simulink model "IOT_Charger"  (R2024b)
settings: Solver=ode23tb  StartTime=0.0  StopTime=1  RelTol=1e-3  EnableMultiTasking=on
PreLoadFcn:
  | % Data of Solar Panel
  | %5000[W]/130[W]
  | % Total power generated by solar panel reaches 5[KW].
  | % each solar panel generates power 130[kW].
  | V = [0    40 80 120 160 180 200 217 240 260 280];
  | I = 5000/130*[0.68 0.675 0.67 0.665 0.660 0.655 0.640 0.6 0.48 0.28 0];
  | 
  | %subplot(211);plot(V,I);xlabel('Voltage[V]');ylabel('Current[a]')
  | %subplot(212);plot(V.*I);title('Power[W]')
  | 
  | % Sample Time[s]
  | Ts =5e-6;
  | 
  | 
  | %MPPT + PV Control
  | % PI control pamameter of Voltage control(Outer loop)
  | Kp_V = 50e-3;
  | Ki_V = 10;
  | 
  | % PI Control pamameter of Current control(Inner loop)
  | Kp_I = 25e-3;
  | Ki_I = 10;
  | 
  | % Utility Interconnection Control
  | % PI Control pamameter of Voltage control(Outer loop)
  | Kp_V2 = 0.01;
  | Ki_V2 = 25;
  | 
  | % PI control pamameter of Current control(Inner loop)
  | Kp_I2 = 0.01;
  | Ki_I2 = 25;
  | 
  | 
  | % Difference of voltege using in MPPT
  | dV = 0.5;
  | 
  | % Battery Control
  | % PI Control pamameter of Voltage control(Outer loop)
  | Kp_VB = 0.4;
  | Ki_VB = 2;
  | 
  | % PI control pamameter of Current control(Inner loop)
  | Kp_IB = 0.1;
  | Ki_IB = 0.5;
undefined symbols (not defined in the file): Ion, Lithium, sigbuilder_block
libraries: spsBreakerLib x120, spsSeriesRLCBranchLib x72, spsBatteryLib x43, spsIdealSwitchLib x29, spsVoltageMeasurementLib x25, spsMosfetLib x19, slpidlib x17, spsSeriesRLCLoadLib x12, spsPWMGeneratorDCDCLib x11, spsCurrentMeasurementLib x10, spsDiodeLib x6, spsPWMGenerator2LevelLib x5
(part 3 of 6)

== system IOT_Charger/Subsystem18/Subsystem20 ==
  Battery : spsBatteryLib/Battery  BatType=Lithium-Ion  NomV=12  NomQ=10  SOC=95  Batt_Tr=30  PresetModel=on  MaxQ=10  MinV=9  FullV=13.9678  Dis_rate=4.3478  R=0.012  Normal_OP=9.0435  expZone="[12.9646     0.491304]"
  Breaker{,1..3} (4 alike) : spsBreakerLib/Breaker  InitialState=0  SwitchingTimes="[1/60  5/60]"  External=on  BreakerResistance=0.01  SnubberResistance=1e6  SnubberCapacitance=inf  Measurements=None  MoreParameters=on  NoBreakLoop=off
  Bus Selector : BusSelector  OutputSignals=SOC (%),Current (A),Voltage (V)
  Scope : Scope  NumInputPorts=3
  Series RLC Branch : spsSeriesRLCBranchLib/Series RLC Branch  LConnTagsString=__new0  RConnTagsString=__new0  BranchType=R  Resistance=1  Inductance=1e-3  SetiL0=off  InitialCurrent=0  Capacitance=1e-6  Setx0=off  InitialVoltage=0  Measurements=None
  + : PMIOPort  Side=Right
  - : PMIOPort  Port=2  Side=Right
  tag scope: s8=global
  wires:
  Battery/1 -> Bus Selector/1
  [c8] -> Breaker3/1, Breaker/1
  Bus Selector/2 -> Scope/2  "<Current (A)>"
  [d8] -> Breaker1/1, Breaker2/1
  Bus Selector/3 -> Scope/3  "<Voltage (V)>"
  Bus Selector/1 -> [s8], Scope/1  "<SOC (%)>"
  connections:
  Breaker2/LConn1 -- Breaker3/RConn1 -- Battery/LConn2
  Breaker1/LConn1 -- Battery/LConn1 -- Breaker/RConn1
  +/RConn1 -- Breaker/LConn1
  Series RLC Branch/LConn1 -- Breaker2/RConn1
  Series RLC Branch/RConn1 -- Breaker1/RConn1
  -/RConn1 -- Breaker3/LConn1

== system IOT_Charger/Subsystem18/Subsystem21 ==
  Battery : spsBatteryLib/Battery  BatType=Lithium-Ion  NomV=12  NomQ=10  SOC=95  Batt_Tr=30  PresetModel=on  MaxQ=10  MinV=9  FullV=13.9678  Dis_rate=4.3478  R=0.012  Normal_OP=9.0435  expZone="[12.9646     0.491304]"
  Breaker{,1..3} (4 alike) : spsBreakerLib/Breaker  InitialState=0  SwitchingTimes="[1/60  5/60]"  External=on  BreakerResistance=0.01  SnubberResistance=1e6  SnubberCapacitance=inf  Measurements=None  MoreParameters=on  NoBreakLoop=off
  Bus Selector : BusSelector  OutputSignals=SOC (%),Current (A),Voltage (V)
  Scope : Scope  NumInputPorts=3
  Series RLC Branch : spsSeriesRLCBranchLib/Series RLC Branch  LConnTagsString=__new0  RConnTagsString=__new0  BranchType=R  Resistance=1  Inductance=1e-3  SetiL0=off  InitialCurrent=0  Capacitance=1e-6  Setx0=off  InitialVoltage=0  Measurements=None
  + : PMIOPort  Side=Right
  - : PMIOPort  Port=2  Side=Right
  tag scope: s7=global
  wires:
  Battery/1 -> Bus Selector/1
  [c7] -> Breaker3/1, Breaker/1
  Bus Selector/2 -> Scope/2  "<Current (A)>"
  [d7] -> Breaker1/1, Breaker2/1
  Bus Selector/3 -> Scope/3  "<Voltage (V)>"
  Bus Selector/1 -> [s7], Scope/1  "<SOC (%)>"
  connections:
  Breaker2/LConn1 -- Breaker3/RConn1 -- Battery/LConn2
  Breaker1/LConn1 -- Battery/LConn1 -- Breaker/RConn1
  +/RConn1 -- Breaker/LConn1
  Series RLC Branch/LConn1 -- Breaker2/RConn1
  Series RLC Branch/RConn1 -- Breaker1/RConn1
  -/RConn1 -- Breaker3/LConn1

== system IOT_Charger/Subsystem18/Subsystem22 ==
  Battery : spsBatteryLib/Battery  BatType=Lithium-Ion  NomV=12  NomQ=10  SOC=95  Batt_Tr=30  PresetModel=on  MaxQ=10  MinV=9  FullV=13.9678  Dis_rate=4.3478  R=0.012  Normal_OP=9.0435  expZone="[12.9646     0.491304]"
  Breaker{,1..3} (4 alike) : spsBreakerLib/Breaker  InitialState=0  SwitchingTimes="[1/60  5/60]"  External=on  BreakerResistance=0.01  SnubberResistance=1e6  SnubberCapacitance=inf  Measurements=None  MoreParameters=on  NoBreakLoop=off
  Bus Selector : BusSelector  OutputSignals=SOC (%),Current (A),Voltage (V)
  Scope : Scope  NumInputPorts=3
  Series RLC Branch : spsSeriesRLCBranchLib/Series RLC Branch  LConnTagsString=__new0  RConnTagsString=__new0  BranchType=R  Resistance=1  Inductance=1e-3  SetiL0=off  InitialCurrent=0  Capacitance=1e-6  Setx0=off  InitialVoltage=0  Measurements=None
  + : PMIOPort  Side=Right
  - : PMIOPort  Port=2  Side=Right
  tag scope: s29=global
  wires:
  Battery/1 -> Bus Selector/1
  [c29] -> Breaker3/1, Breaker/1
  Bus Selector/2 -> Scope/2  "<Current (A)>"
  [d29] -> Breaker1/1, Breaker2/1
  Bus Selector/3 -> Scope/3  "<Voltage (V)>"
  Bus Selector/1 -> [s29], Scope/1  "<SOC (%)>"
  connections:
  Breaker2/LConn1 -- Breaker3/RConn1 -- Battery/LConn2
  Breaker1/LConn1 -- Battery/LConn1 -- Breaker/RConn1
  +/RConn1 -- Breaker/LConn1
  Series RLC Branch/LConn1 -- Breaker2/RConn1
  Series RLC Branch/RConn1 -- Breaker1/RConn1
  -/RConn1 -- Breaker3/LConn1

== system IOT_Charger/Subsystem18/Subsystem23 ==
  Battery : spsBatteryLib/Battery  BatType=Lithium-Ion  NomV=12  NomQ=10  SOC=95  Batt_Tr=30  PresetModel=on  MaxQ=10  MinV=9  FullV=13.9678  Dis_rate=4.3478  R=0.012  Normal_OP=9.0435  expZone="[12.9646     0.491304]"
  Breaker{,1..3} (4 alike) : spsBreakerLib/Breaker  InitialState=0  SwitchingTimes="[1/60  5/60]"  External=on  BreakerResistance=0.01  SnubberResistance=1e6  SnubberCapacitance=inf  Measurements=None  MoreParameters=on  NoBreakLoop=off
  Bus Selector : BusSelector  OutputSignals=SOC (%),Current (A),Voltage (V)
  Scope : Scope  NumInputPorts=3
  Series RLC Branch : spsSeriesRLCBranchLib/Series RLC Branch  LConnTagsString=__new0  RConnTagsString=__new0  BranchType=R  Resistance=1  Inductance=1e-3  SetiL0=off  InitialCurrent=0  Capacitance=1e-6  Setx0=off  InitialVoltage=0  Measurements=None
  + : PMIOPort  Side=Right
  - : PMIOPort  Port=2  Side=Right
  tag scope: s30=global
  wires:
  Battery/1 -> Bus Selector/1
  [c30] -> Breaker3/1, Breaker/1
  Bus Selector/2 -> Scope/2  "<Current (A)>"
  [d30] -> Breaker1/1, Breaker2/1
  Bus Selector/3 -> Scope/3  "<Voltage (V)>"
  Bus Selector/1 -> [s30], Scope/1  "<SOC (%)>"
  connections:
  Breaker2/LConn1 -- Breaker3/RConn1 -- Battery/LConn2
  Breaker1/LConn1 -- Battery/LConn1 -- Breaker/RConn1
  +/RConn1 -- Breaker/LConn1
  Series RLC Branch/LConn1 -- Breaker2/RConn1
  Series RLC Branch/RConn1 -- Breaker1/RConn1
  -/RConn1 -- Breaker3/LConn1

== system IOT_Charger/Subsystem18/Subsystem24 ==
  Battery : spsBatteryLib/Battery  BatType=Lithium-Ion  NomV=12  NomQ=10  SOC=95  Batt_Tr=30  PresetModel=on  MaxQ=10  MinV=9  FullV=13.9678  Dis_rate=4.3478  R=0.012  Normal_OP=9.0435  expZone="[12.9646     0.491304]"
  Breaker{,1..3} (4 alike) : spsBreakerLib/Breaker  InitialState=0  SwitchingTimes="[1/60  5/60]"  External=on  BreakerResistance=0.01  SnubberResistance=1e6  SnubberCapacitance=inf  Measurements=None  MoreParameters=on  NoBreakLoop=off
  Bus Selector : BusSelector  OutputSignals=SOC (%),Current (A),Voltage (V)
  Scope : Scope  NumInputPorts=3
  Series RLC Branch : spsSeriesRLCBranchLib/Series RLC Branch  LConnTagsString=__new0  RConnTagsString=__new0  BranchType=R  Resistance=1  Inductance=1e-3  SetiL0=off  InitialCurrent=0  Capacitance=1e-6  Setx0=off  InitialVoltage=0  Measurements=None
  + : PMIOPort  Side=Right
  - : PMIOPort  Port=2  Side=Right
  tag scope: s26=global
  wires:
  Battery/1 -> Bus Selector/1
  [c26] -> Breaker3/1, Breaker/1
  Bus Selector/2 -> Scope/2  "<Current (A)>"
  [d26] -> Breaker1/1, Breaker2/1
  Bus Selector/3 -> Scope/3  "<Voltage (V)>"
  Bus Selector/1 -> [s26], Scope/1  "<SOC (%)>"
  connections:
  Breaker2/LConn1 -- Breaker3/RConn1 -- Battery/LConn2
  Breaker1/LConn1 -- Battery/LConn1 -- Breaker/RConn1
  +/RConn1 -- Breaker/LConn1
  Series RLC Branch/LConn1 -- Breaker2/RConn1
  Series RLC Branch/RConn1 -- Breaker1/RConn1
  -/RConn1 -- Breaker3/LConn1

== system IOT_Charger/Subsystem18/Subsystem25 ==
  Battery : spsBatteryLib/Battery  BatType=Lithium-Ion  NomV=12  NomQ=10  SOC=95  Batt_Tr=30  PresetModel=on  MaxQ=10  MinV=9  FullV=13.9678  Dis_rate=4.3478  R=0.012  Normal_OP=9.0435  expZone="[12.9646     0.491304]"
  Breaker{,1..3} (4 alike) : spsBreakerLib/Breaker  InitialState=0  SwitchingTimes="[1/60  5/60]"  External=on  BreakerResistance=0.01  SnubberResistance=1e6  SnubberCapacitance=inf  Measurements=None  MoreParameters=on  NoBreakLoop=off
  Bus Selector : BusSelector  OutputSignals=SOC (%),Current (A),Voltage (V)
  Scope : Scope  NumInputPorts=3
  Series RLC Branch : spsSeriesRLCBranchLib/Series RLC Branch  LConnTagsString=__new0  RConnTagsString=__new0  BranchType=R  Resistance=1  Inductance=1e-3  SetiL0=off  InitialCurrent=0  Capacitance=1e-6  Setx0=off  InitialVoltage=0  Measurements=None
  + : PMIOPort  Side=Right
  - : PMIOPort  Port=2  Side=Right
  tag scope: s28=global
  wires:
  Battery/1 -> Bus Selector/1
  [c28] -> Breaker3/1, Breaker/1
  Bus Selector/2 -> Scope/2  "<Current (A)>"
  [d28] -> Breaker1/1, Breaker2/1
  Bus Selector/3 -> Scope/3  "<Voltage (V)>"
  Bus Selector/1 -> [s28], Scope/1  "<SOC (%)>"
  connections:
  Breaker2/LConn1 -- Breaker3/RConn1 -- Battery/LConn2
  Breaker1/LConn1 -- Battery/LConn1 -- Breaker/RConn1
  +/RConn1 -- Breaker/LConn1
  Series RLC Branch/LConn1 -- Breaker2/RConn1
  Series RLC Branch/RConn1 -- Breaker1/RConn1
  -/RConn1 -- Breaker3/LConn1

== system IOT_Charger/Subsystem18/Subsystem26 ==
  Battery : spsBatteryLib/Battery  BatType=Lithium-Ion  NomV=12  NomQ=10  SOC=95  Batt_Tr=30  PresetModel=on  MaxQ=10  MinV=9  FullV=13.9678  Dis_rate=4.3478  R=0.012  Normal_OP=9.0435  expZone="[12.9646     0.491304]"
  Breaker{,1..3} (4 alike) : spsBreakerLib/Breaker  InitialState=0  SwitchingTimes="[1/60  5/60]"  External=on  BreakerResistance=0.01  SnubberResistance=1e6  SnubberCapacitance=inf  Measurements=None  MoreParameters=on  NoBreakLoop=off
  Bus Selector : BusSelector  OutputSignals=SOC (%),Current (A),Voltage (V)
  Scope : Scope  NumInputPorts=3
  Series RLC Branch : spsSeriesRLCBranchLib/Series RLC Branch  LConnTagsString=__new0  RConnTagsString=__new0  BranchType=R  Resistance=1  Inductance=1e-3  SetiL0=off  InitialCurrent=0  Capacitance=1e-6  Setx0=off  InitialVoltage=0  Measurements=None
  + : PMIOPort  Side=Right
  - : PMIOPort  Port=2  Side=Right
  tag scope: s27=global
  wires:
  Battery/1 -> Bus Selector/1
  [c27] -> Breaker3/1, Breaker/1
  Bus Selector/2 -> Scope/2  "<Current (A)>"
  [d27] -> Breaker1/1, Breaker2/1
  Bus Selector/3 -> Scope/3  "<Voltage (V)>"
  Bus Selector/1 -> [s27], Scope/1  "<SOC (%)>"
  connections:
  Breaker2/LConn1 -- Breaker3/RConn1 -- Battery/LConn2
  Breaker1/LConn1 -- Battery/LConn1 -- Breaker/RConn1
  +/RConn1 -- Breaker/LConn1
  Series RLC Branch/LConn1 -- Breaker2/RConn1
  Series RLC Branch/RConn1 -- Breaker1/RConn1
  -/RConn1 -- Breaker3/LConn1

== system IOT_Charger/Subsystem18/Subsystem27 ==
  Battery : spsBatteryLib/Battery  BatType=Lithium-Ion  NomV=12  NomQ=10  SOC=95  Batt_Tr=30  PresetModel=on  MaxQ=10  MinV=9  FullV=13.9678  Dis_rate=4.3478  R=0.012  Normal_OP=9.0435  expZone="[12.9646     0.491304]"
  Breaker{,1..3} (4 alike) : spsBreakerLib/Breaker  InitialState=0  SwitchingTimes="[1/60  5/60]"  External=on  BreakerResistance=0.01  SnubberResistance=1e6  SnubberCapacitance=inf  Measurements=None  MoreParameters=on  NoBreakLoop=off
  Bus Selector : BusSelector  OutputSignals=SOC (%),Current (A),Voltage (V)
  Scope : Scope  NumInputPorts=3
  Series RLC Branch : spsSeriesRLCBranchLib/Series RLC Branch  LConnTagsString=__new0  RConnTagsString=__new0  BranchType=R  Resistance=1  Inductance=1e-3  SetiL0=off  InitialCurrent=0  Capacitance=1e-6  Setx0=off  InitialVoltage=0  Measurements=None
  + : PMIOPort  Side=Right
  - : PMIOPort  Port=2  Side=Right
  tag scope: s24=global
  wires:
  Battery/1 -> Bus Selector/1
  [c24] -> Breaker3/1, Breaker/1
  Bus Selector/2 -> Scope/2  "<Current (A)>"
  [d24] -> Breaker1/1, Breaker2/1
  Bus Selector/3 -> Scope/3  "<Voltage (V)>"
  Bus Selector/1 -> [s24], Scope/1  "<SOC (%)>"
  connections:
  Breaker2/LConn1 -- Breaker3/RConn1 -- Battery/LConn2
  Breaker1/LConn1 -- Battery/LConn1 -- Breaker/RConn1
  +/RConn1 -- Breaker/LConn1
  Series RLC Branch/LConn1 -- Breaker2/RConn1
  Series RLC Branch/RConn1 -- Breaker1/RConn1
  -/RConn1 -- Breaker3/LConn1

== system IOT_Charger/Subsystem18/Subsystem28 ==
  Battery : spsBatteryLib/Battery  BatType=Lithium-Ion  NomV=12  NomQ=10  SOC=95  Batt_Tr=30  PresetModel=on  MaxQ=10  MinV=9  FullV=13.9678  Dis_rate=4.3478  R=0.012  Normal_OP=9.0435  expZone="[12.9646     0.491304]"
  Breaker{,1..3} (4 alike) : spsBreakerLib/Breaker  InitialState=0  SwitchingTimes="[1/60  5/60]"  External=on  BreakerResistance=0.01  SnubberResistance=1e6  SnubberCapacitance=inf  Measurements=None  MoreParameters=on  NoBreakLoop=off
  Bus Selector : BusSelector  OutputSignals=SOC (%),Current (A),Voltage (V)
  Scope : Scope  NumInputPorts=3
  Series RLC Branch : spsSeriesRLCBranchLib/Series RLC Branch  LConnTagsString=__new0  RConnTagsString=__new0  BranchType=R  Resistance=1  Inductance=1e-3  SetiL0=off  InitialCurrent=0  Capacitance=1e-6  Setx0=off  InitialVoltage=0  Measurements=None
  + : PMIOPort  Side=Right
  - : PMIOPort  Port=2  Side=Right
  tag scope: s23=global
  wires:
  Battery/1 -> Bus Selector/1
  [c23] -> Breaker3/1, Breaker/1
  Bus Selector/2 -> Scope/2  "<Current (A)>"
  [d23] -> Breaker1/1, Breaker2/1
  Bus Selector/3 -> Scope/3  "<Voltage (V)>"
  Bus Selector/1 -> [s23], Scope/1  "<SOC (%)>"
  connections:
  Breaker2/LConn1 -- Breaker3/RConn1 -- Battery/LConn2
  Breaker1/LConn1 -- Battery/LConn1 -- Breaker/RConn1
  +/RConn1 -- Breaker/LConn1
  Series RLC Branch/LConn1 -- Breaker2/RConn1
  Series RLC Branch/RConn1 -- Breaker1/RConn1
  -/RConn1 -- Breaker3/LConn1

== system IOT_Charger/Subsystem18/Subsystem29 ==
  Battery : spsBatteryLib/Battery  BatType=Lithium-Ion  NomV=12  NomQ=10  SOC=95  Batt_Tr=30  PresetModel=on  MaxQ=10  MinV=9  FullV=13.9678  Dis_rate=4.3478  R=0.012  Normal_OP=9.0435  expZone="[12.9646     0.491304]"
  Breaker{,1..3} (4 alike) : spsBreakerLib/Breaker  InitialState=0  SwitchingTimes="[1/60  5/60]"  External=on  BreakerResistance=0.01  SnubberResistance=1e6  SnubberCapacitance=inf  Measurements=None  MoreParameters=on  NoBreakLoop=off
  Bus Selector : BusSelector  OutputSignals=SOC (%),Current (A),Voltage (V)
  Scope : Scope  NumInputPorts=3
  Series RLC Branch : spsSeriesRLCBranchLib/Series RLC Branch  LConnTagsString=__new0  RConnTagsString=__new0  BranchType=R  Resistance=1  Inductance=1e-3  SetiL0=off  InitialCurrent=0  Capacitance=1e-6  Setx0=off  InitialVoltage=0  Measurements=None
  + : PMIOPort  Side=Right
  - : PMIOPort  Port=2  Side=Right
  tag scope: s22=global
  wires:
  Battery/1 -> Bus Selector/1
  [c22] -> Breaker3/1, Breaker/1
  Bus Selector/2 -> Scope/2  "<Current (A)>"
  [d22] -> Breaker1/1, Breaker2/1
  Bus Selector/3 -> Scope/3  "<Voltage (V)>"
  Bus Selector/1 -> [s22], Scope/1  "<SOC (%)>"
  connections:
  Breaker2/LConn1 -- Breaker3/RConn1 -- Battery/LConn2
  Breaker1/LConn1 -- Battery/LConn1 -- Breaker/RConn1
  +/RConn1 -- Breaker/LConn1
  Series RLC Branch/LConn1 -- Breaker2/RConn1
  Series RLC Branch/RConn1 -- Breaker1/RConn1
  -/RConn1 -- Breaker3/LConn1

== system IOT_Charger/Subsystem18/Subsystem3 ==
  Battery : spsBatteryLib/Battery  BatType=Lithium-Ion  NomV=12  NomQ=10  SOC=95  Batt_Tr=30  PresetModel=on  MaxQ=10  MinV=9  FullV=13.9678  Dis_rate=4.3478  R=0.012  Normal_OP=9.0435  expZone="[12.9646     0.491304]"
  Breaker{,1..3} (4 alike) : spsBreakerLib/Breaker  InitialState=0  SwitchingTimes="[1/60  5/60]"  External=on  BreakerResistance=0.01  SnubberResistance=1e6  SnubberCapacitance=inf  Measurements=None  MoreParameters=on  NoBreakLoop=off
  Bus Selector : BusSelector  OutputSignals=SOC (%),Current (A),Voltage (V)
  Scope : Scope  NumInputPorts=3
  Series RLC Branch : spsSeriesRLCBranchLib/Series RLC Branch  LConnTagsString=__new0  RConnTagsString=__new0  BranchType=R  Resistance=1  Inductance=1e-3  SetiL0=off  InitialCurrent=0  Capacitance=1e-6  Setx0=off  InitialVoltage=0  Measurements=None
  + : PMIOPort  Side=Right
  - : PMIOPort  Port=2  Side=Right
  tag scope: s4=global
  wires:
  Battery/1 -> Bus Selector/1
  [c4] -> Breaker3/1, Breaker/1
  Bus Selector/2 -> Scope/2  "<Current (A)>"
  [d4] -> Breaker1/1, Breaker2/1
  Bus Selector/3 -> Scope/3  "<Voltage (V)>"
  Bus Selector/1 -> [s4], Scope/1  "<SOC (%)>"
  connections:
  Breaker2/LConn1 -- Breaker3/RConn1 -- Battery/LConn2
  Breaker1/LConn1 -- Battery/LConn1 -- Breaker/RConn1
  +/RConn1 -- Breaker/LConn1
  Series RLC Branch/LConn1 -- Breaker2/RConn1
  Series RLC Branch/RConn1 -- Breaker1/RConn1
  -/RConn1 -- Breaker3/LConn1

== system IOT_Charger/Subsystem18/Subsystem4 ==
  Battery : spsBatteryLib/Battery  BatType=Lithium-Ion  NomV=12  NomQ=10  SOC=95  Batt_Tr=30  PresetModel=on  MaxQ=10  MinV=9  FullV=13.9678  Dis_rate=4.3478  R=0.012  Normal_OP=9.0435  expZone="[12.9646     0.491304]"
  Breaker{,1..3} (4 alike) : spsBreakerLib/Breaker  InitialState=0  SwitchingTimes="[1/60  5/60]"  External=on  BreakerResistance=0.01  SnubberResistance=1e6  SnubberCapacitance=inf  Measurements=None  MoreParameters=on  NoBreakLoop=off
  Bus Selector : BusSelector  OutputSignals=SOC (%),Current (A),Voltage (V)
  Scope : Scope  NumInputPorts=3
  Series RLC Branch : spsSeriesRLCBranchLib/Series RLC Branch  LConnTagsString=__new0  RConnTagsString=__new0  BranchType=R  Resistance=1  Inductance=1e-3  SetiL0=off  InitialCurrent=0  Capacitance=1e-6  Setx0=off  InitialVoltage=0  Measurements=None
  + : PMIOPort  Side=Right
  - : PMIOPort  Port=2  Side=Right
  tag scope: s3=global
  wires:
  Battery/1 -> Bus Selector/1
  [c3] -> Breaker3/1, Breaker/1
  Bus Selector/2 -> Scope/2  "<Current (A)>"
  [d3] -> Breaker1/1, Breaker2/1
  Bus Selector/3 -> Scope/3  "<Voltage (V)>"
  Bus Selector/1 -> [s3], Scope/1  "<SOC (%)>"
  connections:
  Breaker2/LConn1 -- Breaker3/RConn1 -- Battery/LConn2
  Breaker1/LConn1 -- Battery/LConn1 -- Breaker/RConn1
  +/RConn1 -- Breaker/LConn1
  Series RLC Branch/LConn1 -- Breaker2/RConn1
  Series RLC Branch/RConn1 -- Breaker1/RConn1
  -/RConn1 -- Breaker3/LConn1

== system IOT_Charger/Subsystem18/Subsystem5 ==
  Battery : spsBatteryLib/Battery  BatType=Lithium-Ion  NomV=12  NomQ=10  SOC=95  Batt_Tr=30  PresetModel=on  MaxQ=10  MinV=9  FullV=13.9678  Dis_rate=4.3478  R=0.012  Normal_OP=9.0435  expZone="[12.9646     0.491304]"
  Breaker{,1..3} (4 alike) : spsBreakerLib/Breaker  InitialState=0  SwitchingTimes="[1/60  5/60]"  External=on  BreakerResistance=0.01  SnubberResistance=1e6  SnubberCapacitance=inf  Measurements=None  MoreParameters=on  NoBreakLoop=off
  Bus Selector : BusSelector  OutputSignals=SOC (%),Current (A),Voltage (V)
  Scope : Scope  NumInputPorts=3
  Series RLC Branch : spsSeriesRLCBranchLib/Series RLC Branch  LConnTagsString=__new0  RConnTagsString=__new0  BranchType=R  Resistance=1  Inductance=1e-3  SetiL0=off  InitialCurrent=0  Capacitance=1e-6  Setx0=off  InitialVoltage=0  Measurements=None
  + : PMIOPort  Side=Right
  - : PMIOPort  Port=2  Side=Right
  tag scope: s2=global
  wires:
  Battery/1 -> Bus Selector/1
  [c2] -> Breaker3/1, Breaker/1
  Bus Selector/2 -> Scope/2  "<Current (A)>"
  [d2] -> Breaker1/1, Breaker2/1
  Bus Selector/3 -> Scope/3  "<Voltage (V)>"
  Bus Selector/1 -> [s2], Scope/1  "<SOC (%)>"
  connections:
  Breaker2/LConn1 -- Breaker3/RConn1 -- Battery/LConn2
  Breaker1/LConn1 -- Battery/LConn1 -- Breaker/RConn1
  +/RConn1 -- Breaker/LConn1
  Series RLC Branch/LConn1 -- Breaker2/RConn1
  Series RLC Branch/RConn1 -- Breaker1/RConn1
  -/RConn1 -- Breaker3/LConn1

== system IOT_Charger/Subsystem18/Subsystem6 ==
  Battery : spsBatteryLib/Battery  BatType=Lithium-Ion  NomV=12  NomQ=10  SOC=95  Batt_Tr=30  PresetModel=on  MaxQ=10  MinV=9  FullV=13.9678  Dis_rate=4.3478  R=0.012  Normal_OP=9.0435  expZone="[12.9646     0.491304]"
  Breaker{,1..3} (4 alike) : spsBreakerLib/Breaker  InitialState=0  SwitchingTimes="[1/60  5/60]"  External=on  BreakerResistance=0.01  SnubberResistance=1e6  SnubberCapacitance=inf  Measurements=None  MoreParameters=on  NoBreakLoop=off
  Bus Selector : BusSelector  OutputSignals=SOC (%),Current (A),Voltage (V)
  Scope : Scope  NumInputPorts=3
  Series RLC Branch : spsSeriesRLCBranchLib/Series RLC Branch  LConnTagsString=__new0  RConnTagsString=__new0  BranchType=R  Resistance=1  Inductance=1e-3  SetiL0=off  InitialCurrent=0  Capacitance=1e-6  Setx0=off  InitialVoltage=0  Measurements=None
  + : PMIOPort  Side=Right
  - : PMIOPort  Port=2  Side=Right
  tag scope: s15=global
  wires:
  Battery/1 -> Bus Selector/1
  [c15] -> Breaker3/1, Breaker/1
  Bus Selector/2 -> Scope/2  "<Current (A)>"
  [d15] -> Breaker1/1, Breaker2/1
  Bus Selector/3 -> Scope/3  "<Voltage (V)>"
  Bus Selector/1 -> [s15], Scope/1  "<SOC (%)>"
  connections:
  Breaker2/LConn1 -- Breaker3/RConn1 -- Battery/LConn2
  Breaker1/LConn1 -- Battery/LConn1 -- Breaker/RConn1
  +/RConn1 -- Breaker/LConn1
  Series RLC Branch/LConn1 -- Breaker2/RConn1
  Series RLC Branch/RConn1 -- Breaker1/RConn1
  -/RConn1 -- Breaker3/LConn1

== system IOT_Charger/Subsystem18/Subsystem7 ==
  Battery : spsBatteryLib/Battery  BatType=Lithium-Ion  NomV=12  NomQ=10  SOC=95  Batt_Tr=30  PresetModel=on  MaxQ=10  MinV=9  FullV=13.9678  Dis_rate=4.3478  R=0.012  Normal_OP=9.0435  expZone="[12.9646     0.491304]"
  Breaker{,1..3} (4 alike) : spsBreakerLib/Breaker  InitialState=0  SwitchingTimes="[1/60  5/60]"  External=on  BreakerResistance=0.01  SnubberResistance=1e6  SnubberCapacitance=inf  Measurements=None  MoreParameters=on  NoBreakLoop=off
  Bus Selector : BusSelector  OutputSignals=SOC (%),Current (A),Voltage (V)
  Scope : Scope  NumInputPorts=3
  Series RLC Branch : spsSeriesRLCBranchLib/Series RLC Branch  LConnTagsString=__new0  RConnTagsString=__new0  BranchType=R  Resistance=1  Inductance=1e-3  SetiL0=off  InitialCurrent=0  Capacitance=1e-6  Setx0=off  InitialVoltage=0  Measurements=None
  + : PMIOPort  Side=Right
  - : PMIOPort  Port=2  Side=Right
  tag scope: s11=global
  wires:
  Battery/1 -> Bus Selector/1
  [c11] -> Breaker3/1, Breaker/1
  Bus Selector/2 -> Scope/2  "<Current (A)>"
  [d11] -> Breaker1/1, Breaker2/1
  Bus Selector/3 -> Scope/3  "<Voltage (V)>"
  Bus Selector/1 -> [s11], Scope/1  "<SOC (%)>"
  connections:
  Breaker2/LConn1 -- Breaker3/RConn1 -- Battery/LConn2
  Breaker1/LConn1 -- Battery/LConn1 -- Breaker/RConn1
  +/RConn1 -- Breaker/LConn1
  Series RLC Branch/LConn1 -- Breaker2/RConn1
  Series RLC Branch/RConn1 -- Breaker1/RConn1
  -/RConn1 -- Breaker3/LConn1

== system IOT_Charger/Subsystem18/Subsystem8 ==
  Battery : spsBatteryLib/Battery  BatType=Lithium-Ion  NomV=12  NomQ=10  SOC=95  Batt_Tr=30  PresetModel=on  MaxQ=10  MinV=9  FullV=13.9678  Dis_rate=4.3478  R=0.012  Normal_OP=9.0435  expZone="[12.9646     0.491304]"
  Breaker{,1..3} (4 alike) : spsBreakerLib/Breaker  InitialState=0  SwitchingTimes="[1/60  5/60]"  External=on  BreakerResistance=0.01  SnubberResistance=1e6  SnubberCapacitance=inf  Measurements=None  MoreParameters=on  NoBreakLoop=off
  Bus Selector : BusSelector  OutputSignals=SOC (%),Current (A),Voltage (V)
  Scope : Scope  NumInputPorts=3
  Series RLC Branch : spsSeriesRLCBranchLib/Series RLC Branch  LConnTagsString=__new0  RConnTagsString=__new0  BranchType=R  Resistance=1  Inductance=1e-3  SetiL0=off  InitialCurrent=0  Capacitance=1e-6  Setx0=off  InitialVoltage=0  Measurements=None
  + : PMIOPort  Side=Right
  - : PMIOPort  Port=2  Side=Right
  tag scope: s19=global
  wires:
  Battery/1 -> Bus Selector/1
  [c19] -> Breaker3/1, Breaker/1
  Bus Selector/2 -> Scope/2  "<Current (A)>"
  [d19] -> Breaker1/1, Breaker2/1
  Bus Selector/3 -> Scope/3  "<Voltage (V)>"
  Bus Selector/1 -> [s19], Scope/1  "<SOC (%)>"
  connections:
  Breaker2/LConn1 -- Breaker3/RConn1 -- Battery/LConn2
  Breaker1/LConn1 -- Battery/LConn1 -- Breaker/RConn1
  +/RConn1 -- Breaker/LConn1
  Series RLC Branch/LConn1 -- Breaker2/RConn1
  Series RLC Branch/RConn1 -- Breaker1/RConn1
  -/RConn1 -- Breaker3/LConn1

== system IOT_Charger/Subsystem18/Subsystem9 ==
  Battery : spsBatteryLib/Battery  BatType=Lithium-Ion  NomV=12  NomQ=10  SOC=95  Batt_Tr=30  PresetModel=on  MaxQ=10  MinV=9  FullV=13.9678  Dis_rate=4.3478  R=0.012  Normal_OP=9.0435  expZone="[12.9646     0.491304]"
  Breaker{,1..3} (4 alike) : spsBreakerLib/Breaker  InitialState=0  SwitchingTimes="[1/60  5/60]"  External=on  BreakerResistance=0.01  SnubberResistance=1e6  SnubberCapacitance=inf  Measurements=None  MoreParameters=on  NoBreakLoop=off
  Bus Selector : BusSelector  OutputSignals=SOC (%),Current (A),Voltage (V)
  Scope : Scope  NumInputPorts=3
  Series RLC Branch : spsSeriesRLCBranchLib/Series RLC Branch  LConnTagsString=__new0  RConnTagsString=__new0  BranchType=R  Resistance=1  Inductance=1e-3  SetiL0=off  InitialCurrent=0  Capacitance=1e-6  Setx0=off  InitialVoltage=0  Measurements=None
  + : PMIOPort  Side=Right
  - : PMIOPort  Port=2  Side=Right
  tag scope: s20=global
  wires:
  Battery/1 -> Bus Selector/1
  [c20] -> Breaker3/1, Breaker/1
  Bus Selector/2 -> Scope/2  "<Current (A)>"
  [d20] -> Breaker1/1, Breaker2/1
  Bus Selector/3 -> Scope/3  "<Voltage (V)>"
  Bus Selector/1 -> [s20], Scope/1  "<SOC (%)>"
  connections:
  Breaker2/LConn1 -- Breaker3/RConn1 -- Battery/LConn2
  Breaker1/LConn1 -- Battery/LConn1 -- Breaker/RConn1
  +/RConn1 -- Breaker/LConn1
  Series RLC Branch/LConn1 -- Breaker2/RConn1
  Series RLC Branch/RConn1 -- Breaker1/RConn1
  -/RConn1 -- Breaker3/LConn1

== system IOT_Charger/Subsystem2/Control ==
  Add : Sum  Inputs=+-
  Add1 : Sum  Inputs=+-
  Constant : Constant  Value=25.99
  Gain : Gain  Gain=-1
  NOT : Logic  Operator=NOT  IconShape=distinctive  AllPortsSameDT=off  OutDataTypeStr=boolean
  PID Controller : slpidlib/PID Controller  Controller=PI  Form=Parallel  TimeDomain=Continuous-time  UseExternalTs=off  SampleTime=-1  IntegratorMethod=Forward Euler  FilterMethod=Forward Euler  ControllerParametersSource=internal  P=0.005  I=10  UseKiTs=off  D=0  UseExternalDerivativeSource=off  N=100  UseFilter=on  TunerSelectOption=Transfer Function Based (PID Tuner App)  InitialConditionSource=internal  InitialConditionForIntegrator=0.54  InitialConditionForFilter=0  DifferentiatorICPrevScaledInput=0  ExternalReset=none  TrackingMode=off  Kt=1  LimitOutput=on  SatLimitsSource=internal  UpperSaturationLimit=0.975  LowerSaturationLimit=0  LinearizeAsGain=on  AntiWindupMode=none  Kb=1  LimitIntegrator=off  UpperIntegratorSaturationLimit=inf  LowerIntegratorSaturationLimit=-inf  POutMin=[]  POutMax=[]  IOutMin=[]  IOutMax=[]  DOutMin=[]  DOutMax=[]  NOutMin=[]  NOutMax=[]  SumOutMin=[]  SumOutMax=[]  SaturationOutMin=[]  SaturationOutMax=[]  PParamMin=[]  PParamMax=[]  IParamMin=[]  IParamMax=[]  DParamMin=[]  DParamMax=[]  NParamMin=[]  NParamMax=[]  KbParamMin=[]  KbParamMax=[]  KtParamMin=[]  KtParamMax=[]  KbOutMin=[]  KbOutMax=[]  KtOutMin=[]  KtOutMax=[]  IntegratorOutMin=[]  IntegratorOutMax=[]  FilterOutMin=[]  FilterOutMax=[]  SumI1OutMin=[]  SumI1OutMax=[]  SumI2OutMin=[]  SumI2OutMax=[]  SumI3OutMin=[]  SumI3OutMax=[]  SumI4OutMin=[]  SumI4OutMax=[]  SumDOutMin=[]  SumDOutMax=[]  DifferentiatorOutMin=[]  DifferentiatorOutMax=[]  FilterDiffOutCoefMin=[]  FilterDiffOutCoefMax=[]  ReciprocalOutMin=[]  ReciprocalOutMax=[]  SumDenOutMin=[]  SumDenOutMax=[]  SumNumOutMin=[]  SumNumOutMax=[]  DivideOutMin=[]  DivideOutMax=[]  UdiffTsProdOutMin=[]  UdiffTsProdOutMax=[]  NTsProdOutMin=[]  NTsProdOutMax=[]  UintegralTsProdOutMin=[]  UintegralTsProdOutMax=[]  UngainTsProdOutMin=[]  UngainTsProdOutMax=[]  ClampingZeroOutDataTypeStr=Inherit: Inherit via back propagation  ClampingZeroOutMin=[]  ClampingZeroOutMax=[]  FilterDenConstantOutDataTypeStr=Inherit: Inherit via back propagation  FilterDenConstantOutMin=[]  FilterDenConstantOutMax=[]  PCopyOutDataTypeStr=Inherit: Inherit via back propagation  PCopyOutMin=[]  PCopyOutMax=[]  NCopyOutDataTypeStr=Inherit: Inherit via back propagation  NCopyOutMin=[]  NCopyOutMax=[]  IntegratorContinuousStateAttributes=''  IntegratorStateMustResolveToSignalObject=off  IntegratorRTWStateStorageClass=Auto  FilterContinuousStateAttributes=''  FilterStateMustResolveToSignalObject=off  FilterRTWStateStorageClass=Auto  ParallelPVariant=InternalParameters  IdealPVariant=Disabled  IVariant=InternalParameters  DVariant=Disabled  IntegratorVariant=Continuous  SatVariant=Enabled  AWVariant=Passthrough  PCopyVariant=Disabled  TRVariant=Disabled  FdbkBlocksVariant=Forward  IdealPFdbkVariant=Disabled  SatFdbkVariant=Disabled  DerivativeFilterVariant=Disabled  NVariant=Disabled  NCopyVariant=Disabled_SignalSpec  FilterICVariant=Disabled  IntegratorICVariant=InternalICs  ExternalResetVariant=Disabled  TRSumVariant=Passthrough  SumFdbkVariant=Disabled  SumVariant=Sum_PI  TsampFilterVariant=InternalTs  TsampNgainVariant=Passthrough  TsampIntegralVariant=Disabled_SignalSpec  ExternalSaturationOutDataTypeStr=Inherit: Same as second input  DerivativeSourceVariant=Disabled  PreIntVariant=InternalPreInt
  PID Controller1 : slpidlib/PID Controller  Controller=PI  Form=Parallel  TimeDomain=Continuous-time  UseExternalTs=off  SampleTime=-1  IntegratorMethod=Forward Euler  FilterMethod=Forward Euler  ControllerParametersSource=internal  P=40  I=2000  UseKiTs=off  D=0  UseExternalDerivativeSource=off  N=100  UseFilter=on  TunerSelectOption=Transfer Function Based (PID Tuner App)  InitialConditionSource=internal  InitialConditionForIntegrator=0.54  InitialConditionForFilter=0  DifferentiatorICPrevScaledInput=0  ExternalReset=none  TrackingMode=off  Kt=1  LimitOutput=on  SatLimitsSource=internal  UpperSaturationLimit=17.39  LowerSaturationLimit=0  LinearizeAsGain=on  AntiWindupMode=none  Kb=1  LimitIntegrator=off  UpperIntegratorSaturationLimit=inf  LowerIntegratorSaturationLimit=-inf  POutMin=[]  POutMax=[]  IOutMin=[]  IOutMax=[]  DOutMin=[]  DOutMax=[]  NOutMin=[]  NOutMax=[]  SumOutMin=[]  SumOutMax=[]  SaturationOutMin=[]  SaturationOutMax=[]  PParamMin=[]  PParamMax=[]  IParamMin=[]  IParamMax=[]  DParamMin=[]  DParamMax=[]  NParamMin=[]  NParamMax=[]  KbParamMin=[]  KbParamMax=[]  KtParamMin=[]  KtParamMax=[]  KbOutMin=[]  KbOutMax=[]  KtOutMin=[]  KtOutMax=[]  IntegratorOutMin=[]  IntegratorOutMax=[]  FilterOutMin=[]  FilterOutMax=[]  SumI1OutMin=[]  SumI1OutMax=[]  SumI2OutMin=[]  SumI2OutMax=[]  SumI3OutMin=[]  SumI3OutMax=[]  SumI4OutMin=[]  SumI4OutMax=[]  SumDOutMin=[]  SumDOutMax=[]  DifferentiatorOutMin=[]  DifferentiatorOutMax=[]  FilterDiffOutCoefMin=[]  FilterDiffOutCoefMax=[]  ReciprocalOutMin=[]  ReciprocalOutMax=[]  SumDenOutMin=[]  SumDenOutMax=[]  SumNumOutMin=[]  SumNumOutMax=[]  DivideOutMin=[]  DivideOutMax=[]  UdiffTsProdOutMin=[]  UdiffTsProdOutMax=[]  NTsProdOutMin=[]  NTsProdOutMax=[]  UintegralTsProdOutMin=[]  UintegralTsProdOutMax=[]  UngainTsProdOutMin=[]  UngainTsProdOutMax=[]  ClampingZeroOutDataTypeStr=Inherit: Inherit via back propagation  ClampingZeroOutMin=[]  ClampingZeroOutMax=[]  FilterDenConstantOutDataTypeStr=Inherit: Inherit via back propagation  FilterDenConstantOutMin=[]  FilterDenConstantOutMax=[]  PCopyOutDataTypeStr=Inherit: Inherit via back propagation  PCopyOutMin=[]  PCopyOutMax=[]  NCopyOutDataTypeStr=Inherit: Inherit via back propagation  NCopyOutMin=[]  NCopyOutMax=[]  IntegratorContinuousStateAttributes=''  IntegratorStateMustResolveToSignalObject=off  IntegratorRTWStateStorageClass=Auto  FilterContinuousStateAttributes=''  FilterStateMustResolveToSignalObject=off  FilterRTWStateStorageClass=Auto  ParallelPVariant=InternalParameters  IdealPVariant=Disabled  IVariant=InternalParameters  DVariant=Disabled  IntegratorVariant=Continuous  SatVariant=Enabled  AWVariant=Passthrough  PCopyVariant=Disabled  TRVariant=Disabled  FdbkBlocksVariant=Forward  IdealPFdbkVariant=Disabled  SatFdbkVariant=Disabled  DerivativeFilterVariant=Disabled  NVariant=Disabled  NCopyVariant=Disabled_SignalSpec  FilterICVariant=Disabled  IntegratorICVariant=InternalICs  ExternalResetVariant=Disabled  TRSumVariant=Passthrough  SumFdbkVariant=Disabled  SumVariant=Sum_PI  TsampFilterVariant=InternalTs  TsampNgainVariant=Passthrough  TsampIntegralVariant=Disabled_SignalSpec  ExternalSaturationOutDataTypeStr=Inherit: Same as second input  DerivativeSourceVariant=Disabled  PreIntVariant=InternalPreInt
  PWM Generator (DC-DC) : spsPWMGeneratorDCDCLib/PWM Generator (DC-DC)  Fsw=10e3  Ts=5e-6
  tag scope: Mosfet_333=global, Mosfet_33=global
  wires:
  Add/1 -> PID Controller/1
  PWM Generator (DC-DC)/1 -> NOT/1, [Mosfet_33]
  PID Controller/1 -> PWM Generator (DC-DC)/1
  NOT/1 -> [Mosfet_333]
  [Ref_Current] -> Add/2
  [Current] -> Add/1
  PID Controller1/1 -> Gain/1
  Gain/1 -> [Ref_Current]
  Add1/1 -> PID Controller1/1
  Constant/1 -> Add1/1
  [Voltage] -> Add1/2

== system IOT_Charger/Subsystem3/Control ==
  Add : Sum  Inputs=+-
  Add1 : Sum  Inputs=+-
  Constant : Constant  Value=25.99
  Gain : Gain  Gain=-1
  NOT : Logic  Operator=NOT  IconShape=distinctive  AllPortsSameDT=off  OutDataTypeStr=boolean
  PID Controller : slpidlib/PID Controller  Controller=PI  Form=Parallel  TimeDomain=Continuous-time  UseExternalTs=off  SampleTime=-1  IntegratorMethod=Forward Euler  FilterMethod=Forward Euler  ControllerParametersSource=internal  P=0.005  I=10  UseKiTs=off  D=0  UseExternalDerivativeSource=off  N=100  UseFilter=on  TunerSelectOption=Transfer Function Based (PID Tuner App)  InitialConditionSource=internal  InitialConditionForIntegrator=0.54  InitialConditionForFilter=0  DifferentiatorICPrevScaledInput=0  ExternalReset=none  TrackingMode=off  Kt=1  LimitOutput=on  SatLimitsSource=internal  UpperSaturationLimit=0.975  LowerSaturationLimit=0  LinearizeAsGain=on  AntiWindupMode=none  Kb=1  LimitIntegrator=off  UpperIntegratorSaturationLimit=inf  LowerIntegratorSaturationLimit=-inf  POutMin=[]  POutMax=[]  IOutMin=[]  IOutMax=[]  DOutMin=[]  DOutMax=[]  NOutMin=[]  NOutMax=[]  SumOutMin=[]  SumOutMax=[]  SaturationOutMin=[]  SaturationOutMax=[]  PParamMin=[]  PParamMax=[]  IParamMin=[]  IParamMax=[]  DParamMin=[]  DParamMax=[]  NParamMin=[]  NParamMax=[]  KbParamMin=[]  KbParamMax=[]  KtParamMin=[]  KtParamMax=[]  KbOutMin=[]  KbOutMax=[]  KtOutMin=[]  KtOutMax=[]  IntegratorOutMin=[]  IntegratorOutMax=[]  FilterOutMin=[]  FilterOutMax=[]  SumI1OutMin=[]  SumI1OutMax=[]  SumI2OutMin=[]  SumI2OutMax=[]  SumI3OutMin=[]  SumI3OutMax=[]  SumI4OutMin=[]  SumI4OutMax=[]  SumDOutMin=[]  SumDOutMax=[]  DifferentiatorOutMin=[]  DifferentiatorOutMax=[]  FilterDiffOutCoefMin=[]  FilterDiffOutCoefMax=[]  ReciprocalOutMin=[]  ReciprocalOutMax=[]  SumDenOutMin=[]  SumDenOutMax=[]  SumNumOutMin=[]  SumNumOutMax=[]  DivideOutMin=[]  DivideOutMax=[]  UdiffTsProdOutMin=[]  UdiffTsProdOutMax=[]  NTsProdOutMin=[]  NTsProdOutMax=[]  UintegralTsProdOutMin=[]  UintegralTsProdOutMax=[]  UngainTsProdOutMin=[]  UngainTsProdOutMax=[]  ClampingZeroOutDataTypeStr=Inherit: Inherit via back propagation  ClampingZeroOutMin=[]  ClampingZeroOutMax=[]  FilterDenConstantOutDataTypeStr=Inherit: Inherit via back propagation  FilterDenConstantOutMin=[]  FilterDenConstantOutMax=[]  PCopyOutDataTypeStr=Inherit: Inherit via back propagation  PCopyOutMin=[]  PCopyOutMax=[]  NCopyOutDataTypeStr=Inherit: Inherit via back propagation  NCopyOutMin=[]  NCopyOutMax=[]  IntegratorContinuousStateAttributes=''  IntegratorStateMustResolveToSignalObject=off  IntegratorRTWStateStorageClass=Auto  FilterContinuousStateAttributes=''  FilterStateMustResolveToSignalObject=off  FilterRTWStateStorageClass=Auto  ParallelPVariant=InternalParameters  IdealPVariant=Disabled  IVariant=InternalParameters  DVariant=Disabled  IntegratorVariant=Continuous  SatVariant=Enabled  AWVariant=Passthrough  PCopyVariant=Disabled  TRVariant=Disabled  FdbkBlocksVariant=Forward  IdealPFdbkVariant=Disabled  SatFdbkVariant=Disabled  DerivativeFilterVariant=Disabled  NVariant=Disabled  NCopyVariant=Disabled_SignalSpec  FilterICVariant=Disabled  IntegratorICVariant=InternalICs  ExternalResetVariant=Disabled  TRSumVariant=Passthrough  SumFdbkVariant=Disabled  SumVariant=Sum_PI  TsampFilterVariant=InternalTs  TsampNgainVariant=Passthrough  TsampIntegralVariant=Disabled_SignalSpec  ExternalSaturationOutDataTypeStr=Inherit: Same as second input  DerivativeSourceVariant=Disabled  PreIntVariant=InternalPreInt
  PID Controller1 : slpidlib/PID Controller  Controller=PI  Form=Parallel  TimeDomain=Continuous-time  UseExternalTs=off  SampleTime=-1  IntegratorMethod=Forward Euler  FilterMethod=Forward Euler  ControllerParametersSource=internal  P=40  I=2000  UseKiTs=off  D=0  UseExternalDerivativeSource=off  N=100  UseFilter=on  TunerSelectOption=Transfer Function Based (PID Tuner App)  InitialConditionSource=internal  InitialConditionForIntegrator=0.54  InitialConditionForFilter=0  DifferentiatorICPrevScaledInput=0  ExternalReset=none  TrackingMode=off  Kt=1  LimitOutput=on  SatLimitsSource=internal  UpperSaturationLimit=17.39  LowerSaturationLimit=0  LinearizeAsGain=on  AntiWindupMode=none  Kb=1  LimitIntegrator=off  UpperIntegratorSaturationLimit=inf  LowerIntegratorSaturationLimit=-inf  POutMin=[]  POutMax=[]  IOutMin=[]  IOutMax=[]  DOutMin=[]  DOutMax=[]  NOutMin=[]  NOutMax=[]  SumOutMin=[]  SumOutMax=[]  SaturationOutMin=[]  SaturationOutMax=[]  PParamMin=[]  PParamMax=[]  IParamMin=[]  IParamMax=[]  DParamMin=[]  DParamMax=[]  NParamMin=[]  NParamMax=[]  KbParamMin=[]  KbParamMax=[]  KtParamMin=[]  KtParamMax=[]  KbOutMin=[]  KbOutMax=[]  KtOutMin=[]  KtOutMax=[]  IntegratorOutMin=[]  IntegratorOutMax=[]  FilterOutMin=[]  FilterOutMax=[]  SumI1OutMin=[]  SumI1OutMax=[]  SumI2OutMin=[]  SumI2OutMax=[]  SumI3OutMin=[]  SumI3OutMax=[]  SumI4OutMin=[]  SumI4OutMax=[]  SumDOutMin=[]  SumDOutMax=[]  DifferentiatorOutMin=[]  DifferentiatorOutMax=[]  FilterDiffOutCoefMin=[]  FilterDiffOutCoefMax=[]  ReciprocalOutMin=[]  ReciprocalOutMax=[]  SumDenOutMin=[]  SumDenOutMax=[]  SumNumOutMin=[]  SumNumOutMax=[]  DivideOutMin=[]  DivideOutMax=[]  UdiffTsProdOutMin=[]  UdiffTsProdOutMax=[]  NTsProdOutMin=[]  NTsProdOutMax=[]  UintegralTsProdOutMin=[]  UintegralTsProdOutMax=[]  UngainTsProdOutMin=[]  UngainTsProdOutMax=[]  ClampingZeroOutDataTypeStr=Inherit: Inherit via back propagation  ClampingZeroOutMin=[]  ClampingZeroOutMax=[]  FilterDenConstantOutDataTypeStr=Inherit: Inherit via back propagation  FilterDenConstantOutMin=[]  FilterDenConstantOutMax=[]  PCopyOutDataTypeStr=Inherit: Inherit via back propagation  PCopyOutMin=[]  PCopyOutMax=[]  NCopyOutDataTypeStr=Inherit: Inherit via back propagation  NCopyOutMin=[]  NCopyOutMax=[]  IntegratorContinuousStateAttributes=''  IntegratorStateMustResolveToSignalObject=off  IntegratorRTWStateStorageClass=Auto  FilterContinuousStateAttributes=''  FilterStateMustResolveToSignalObject=off  FilterRTWStateStorageClass=Auto  ParallelPVariant=InternalParameters  IdealPVariant=Disabled  IVariant=InternalParameters  DVariant=Disabled  IntegratorVariant=Continuous  SatVariant=Enabled  AWVariant=Passthrough  PCopyVariant=Disabled  TRVariant=Disabled  FdbkBlocksVariant=Forward  IdealPFdbkVariant=Disabled  SatFdbkVariant=Disabled  DerivativeFilterVariant=Disabled  NVariant=Disabled  NCopyVariant=Disabled_SignalSpec  FilterICVariant=Disabled  IntegratorICVariant=InternalICs  ExternalResetVariant=Disabled  TRSumVariant=Passthrough  SumFdbkVariant=Disabled  SumVariant=Sum_PI  TsampFilterVariant=InternalTs  TsampNgainVariant=Passthrough  TsampIntegralVariant=Disabled_SignalSpec  ExternalSaturationOutDataTypeStr=Inherit: Same as second input  DerivativeSourceVariant=Disabled  PreIntVariant=InternalPreInt
  PWM Generator (DC-DC) : spsPWMGeneratorDCDCLib/PWM Generator (DC-DC)  Fsw=10e3  Ts=5e-6
  tag scope: Mosfet_444=global, Mosfet_44=global
  wires:
  Add/1 -> PID Controller/1
  PWM Generator (DC-DC)/1 -> NOT/1, [Mosfet_44]
  PID Controller/1 -> PWM Generator (DC-DC)/1
  NOT/1 -> [Mosfet_444]
  [Ref_Current] -> Add/2
  [Current] -> Add/1
  PID Controller1/1 -> Gain/1
  Gain/1 -> [Ref_Current]
  Add1/1 -> PID Controller1/1
  Constant/1 -> Add1/1
  [Voltage] -> Add1/2

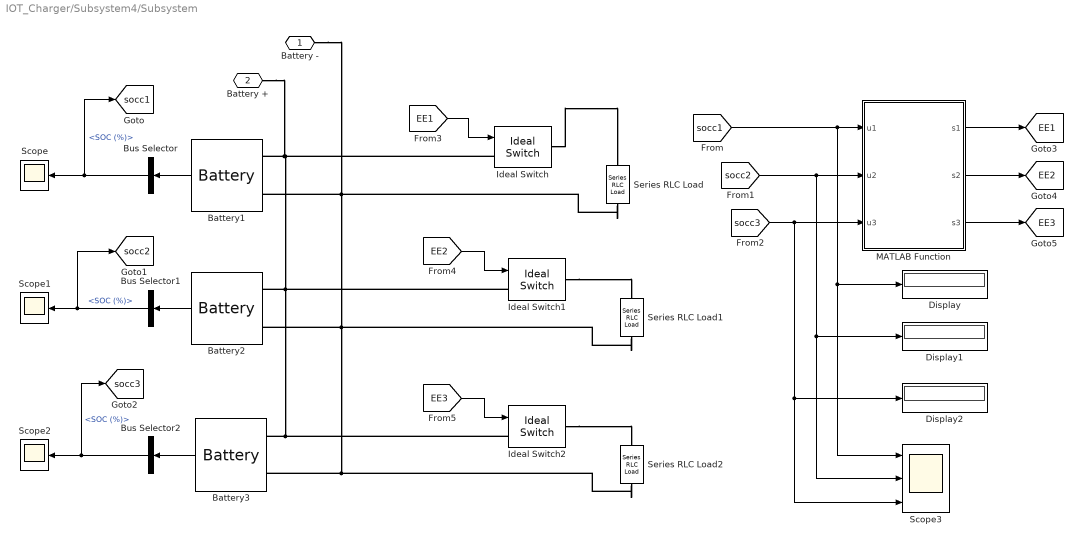
== system IOT_Charger/Subsystem4/Subsystem ==
  Battery1 : spsBatteryLib/Battery  BatType=Lithium-Ion  NomV=3.6  NomQ=4  SOC=100  Batt_Tr=1  PresetModel=on  MaxQ=4  MinV=2.7  FullV=4.1904  Dis_rate=1.7391  R=0.009  Normal_OP=3.6174  expZone="[3.8894     0.19652]"
  Battery2 : spsBatteryLib/Battery  BatType=Lithium-Ion  NomV=3.6  NomQ=4  SOC=60  Batt_Tr=1  PresetModel=on  MaxQ=4  MinV=2.7  FullV=4.1904  Dis_rate=1.7391  R=0.009  Normal_OP=3.6174  expZone="[3.8894     0.19652]"
  Battery3 : spsBatteryLib/Battery  BatType=Lithium-Ion  NomV=3.6  NomQ=4  SOC=30  Batt_Tr=1  PresetModel=on  MaxQ=4  MinV=2.7  FullV=4.1904  Dis_rate=1.7391  R=0.009  Normal_OP=3.6174  expZone="[3.8894     0.19652]"
  Bus Selector : BusSelector  OutputSignals=SOC (%)
  Bus Selector1 : BusSelector  OutputSignals=SOC (%)
  Bus Selector2 : BusSelector  OutputSignals=SOC (%)
  Display : Display
  Display1 : Display
  Display2 : Display
  Ideal Switch : spsIdealSwitchLib/Ideal Switch  Ron=0.001  Lon=0  IC=0  Rs=1e5  Cs=inf  Measurements=off
  Ideal Switch1 : spsIdealSwitchLib/Ideal Switch  Ron=0.001  Lon=0  IC=0  Rs=1e5  Cs=inf  Measurements=off
  Ideal Switch2 : spsIdealSwitchLib/Ideal Switch  Ron=0.001  Lon=0  IC=0  Rs=1e5  Cs=inf  Measurements=off
  MATLAB Function : MATLAB Function  TreatAsAtomicUnit=on
  Scope : Scope
  Scope1 : Scope
  Scope2 : Scope
  Scope3 : Scope  NumInputPorts=3
  Series RLC Load : spsSeriesRLCLoadLib/Series RLC Load  LConnTagsString=a  RConnTagsString=__new0  NominalVoltage=1000  NominalFrequency=60  ActivePower=10e3  InductivePower=0  CapacitivePower=0  Setx0=off  InitialVoltage=0  SetiL0=off  InitialCurrent=0  Measurements=None  LoadType=constant Z
  Series RLC Load1 : spsSeriesRLCLoadLib/Series RLC Load  LConnTagsString=a  RConnTagsString=__new0  NominalVoltage=1000  NominalFrequency=60  ActivePower=10e3  InductivePower=0  CapacitivePower=0  Setx0=off  InitialVoltage=0  SetiL0=off  InitialCurrent=0  Measurements=None  LoadType=constant Z
  Series RLC Load2 : spsSeriesRLCLoadLib/Series RLC Load  LConnTagsString=a  RConnTagsString=__new0  NominalVoltage=1000  NominalFrequency=60  ActivePower=10e3  InductivePower=0  CapacitivePower=0  Setx0=off  InitialVoltage=0  SetiL0=off  InitialCurrent=0  Measurements=None  LoadType=constant Z
  Battery - : PMIOPort  Side=Left
  Battery + : PMIOPort  Port=2  Side=Left
  tag scope: EE1=global, EE2=global, EE3=global, socc1=global, socc2=global, socc3=global
  wires:
  Battery2/1 -> Bus Selector1/1
  Bus Selector/1 -> [socc1], Scope/1  "<SOC (%)>"
  [EE3] -> Ideal Switch2/1
  Bus Selector2/1 -> [socc3], Scope2/1  "<SOC (%)>"
  Bus Selector1/1 -> [socc2], Scope1/1  "<SOC (%)>"
  Battery3/1 -> Bus Selector2/1
  [socc2] -> MATLAB Function/2(u2), Display1/1, Scope3/2
  [socc1] -> Display/1, Scope3/1, MATLAB Function/1(u1)
  Battery1/1 -> Bus Selector/1
  [socc3] -> Display2/1, Scope3/3, MATLAB Function/3(u3)
  MATLAB Function/2(s2) -> [EE2]
  MATLAB Function/3(s3) -> [EE3]
  MATLAB Function/1(s1) -> [EE1]
  [EE1] -> Ideal Switch/1
  [EE2] -> Ideal Switch1/1
  connections:
  Series RLC Load/RConn1 -- Battery3/LConn2 -- Series RLC Load2/RConn1 -- Battery2/LConn2 -- Series RLC Load1/RConn1 -- Battery -/RConn1 -- Battery1/LConn2
  Ideal Switch1/RConn1 -- Series RLC Load1/LConn1
  Ideal Switch2/RConn1 -- Series RLC Load2/LConn1
  Ideal Switch/RConn1 -- Series RLC Load/LConn1
  Ideal Switch/LConn1 -- Battery +/RConn1 -- Battery1/LConn1 -- Battery3/LConn1 -- Ideal Switch2/LConn1 -- Battery2/LConn1 -- Ideal Switch1/LConn1

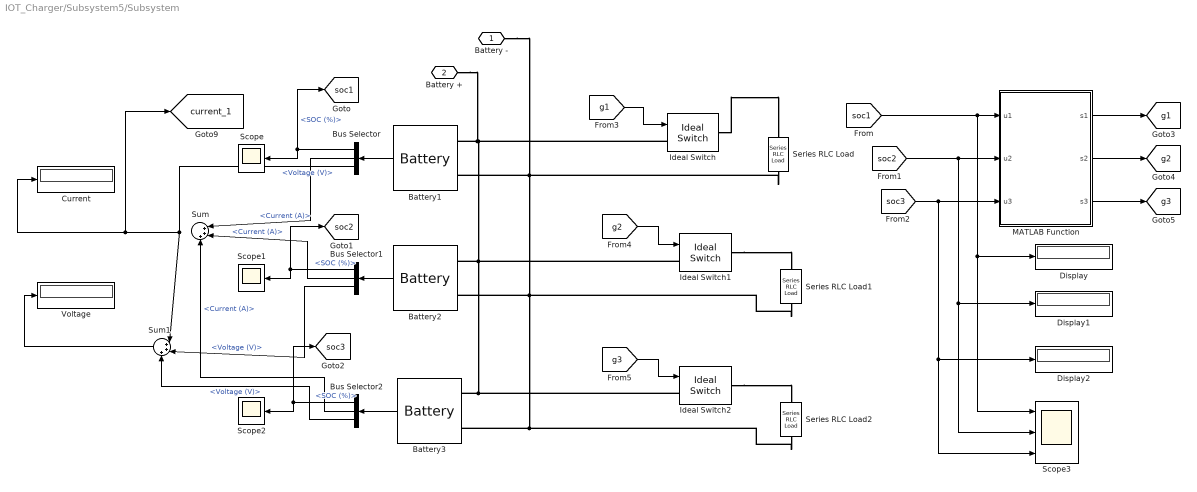
== system IOT_Charger/Subsystem5/Subsystem ==
  Battery1 : spsBatteryLib/Battery  BatType=Lithium-Ion  NomV=12  NomQ=100  SOC=100  Batt_Tr=1  PresetModel=on  MaxQ=100  MinV=9  FullV=13.9678  Dis_rate=43.4783  R=0.0012  Normal_OP=90.4348  expZone="[12.9646      4.91304]"
  Battery2 : spsBatteryLib/Battery  BatType=Lithium-Ion  NomV=12  NomQ=100  SOC=60  Batt_Tr=1  PresetModel=on  MaxQ=100  MinV=9  FullV=13.9678  Dis_rate=43.4783  R=0.0012  Normal_OP=90.4348  expZone="[12.9646      4.91304]"
  Battery3 : spsBatteryLib/Battery  BatType=Lithium-Ion  NomV=12  NomQ=100  SOC=30  Batt_Tr=1  PresetModel=on  MaxQ=100  MinV=9  FullV=13.9678  Dis_rate=43.4783  R=0.0012  Normal_OP=90.4348  expZone="[12.9646      4.91304]"
  Bus Selector : BusSelector  OutputSignals=SOC (%),Current (A),Voltage (V)
  Bus Selector1 : BusSelector  OutputSignals=SOC (%),Current (A),Voltage (V)
  Bus Selector2 : BusSelector  OutputSignals=SOC (%),Current (A),Voltage (V)
  Current : Display
  Display : Display
  Display1 : Display
  Display2 : Display
  Ideal Switch : spsIdealSwitchLib/Ideal Switch  Ron=0.001  Lon=0  IC=0  Rs=1e5  Cs=inf  Measurements=off
  Ideal Switch1 : spsIdealSwitchLib/Ideal Switch  Ron=0.001  Lon=0  IC=0  Rs=1e5  Cs=inf  Measurements=off
  Ideal Switch2 : spsIdealSwitchLib/Ideal Switch  Ron=0.001  Lon=0  IC=0  Rs=1e5  Cs=inf  Measurements=off
  MATLAB Function : MATLAB Function  TreatAsAtomicUnit=on
  Scope : Scope
  Scope1 : Scope
  Scope2 : Scope
  Scope3 : Scope  NumInputPorts=3
  Series RLC Load : spsSeriesRLCLoadLib/Series RLC Load  LConnTagsString=a  RConnTagsString=__new0  NominalVoltage=1000  NominalFrequency=60  ActivePower=10e3  InductivePower=0  CapacitivePower=0  Setx0=off  InitialVoltage=0  SetiL0=off  InitialCurrent=0  Measurements=None  LoadType=constant Z
  Series RLC Load1 : spsSeriesRLCLoadLib/Series RLC Load  LConnTagsString=a  RConnTagsString=__new0  NominalVoltage=1000  NominalFrequency=60  ActivePower=10e3  InductivePower=0  CapacitivePower=0  Setx0=off  InitialVoltage=0  SetiL0=off  InitialCurrent=0  Measurements=None  LoadType=constant Z
  Series RLC Load2 : spsSeriesRLCLoadLib/Series RLC Load  LConnTagsString=a  RConnTagsString=__new0  NominalVoltage=1000  NominalFrequency=60  ActivePower=10e3  InductivePower=0  CapacitivePower=0  Setx0=off  InitialVoltage=0  SetiL0=off  InitialCurrent=0  Measurements=None  LoadType=constant Z
  Sum : Sum  Inputs=|+++
  Sum1 : Sum  Inputs=|+++
  Voltage : Display
  Battery - : PMIOPort  Side=Left
  Battery + : PMIOPort  Port=2  Side=Left
  tag scope: current_1=global, g1=global, g2=global, g3=global, soc1=global, soc2=global, soc3=global
  wires:
  Battery2/1 -> Bus Selector1/1
  Bus Selector/1 -> Scope/1, [soc1]  "<SOC (%)>"
  [g3] -> Ideal Switch2/1
  Bus Selector2/1 -> Scope2/1, [soc3]  "<SOC (%)>"
  Bus Selector1/1 -> Scope1/1, [soc2]  "<SOC (%)>"
  Battery3/1 -> Bus Selector2/1
  [soc2] -> MATLAB Function/2(u2), Display1/1, Scope3/2
  [soc1] -> Display/1, Scope3/1, MATLAB Function/1(u1)
  Battery1/1 -> Bus Selector/1
  [soc3] -> Display2/1, Scope3/3, MATLAB Function/3(u3)
  MATLAB Function/2(s2) -> [g2]
  MATLAB Function/3(s3) -> [g3]
  MATLAB Function/1(s1) -> [g1]
  [g1] -> Ideal Switch/1
  [g2] -> Ideal Switch1/1
  Bus Selector/2 -> Sum/1  "<Current (A)>"
  Bus Selector1/2 -> Sum/2  "<Current (A)>"
  Bus Selector2/2 -> Sum/3  "<Current (A)>"
  Bus Selector/3 -> [current_1], Current/1, Sum1/1  "<Voltage (V)>"
  Bus Selector1/3 -> Sum1/2  "<Voltage (V)>"
  Bus Selector2/3 -> Sum1/3  "<Voltage (V)>"
  Sum1/1 -> Voltage/1
  connections:
  Series RLC Load/RConn1 -- Battery3/LConn2 -- Series RLC Load2/RConn1 -- Battery2/LConn2 -- Series RLC Load1/RConn1 -- Battery -/RConn1 -- Battery1/LConn2
  Ideal Switch1/RConn1 -- Series RLC Load1/LConn1
  Ideal Switch2/RConn1 -- Series RLC Load2/LConn1
  Ideal Switch/RConn1 -- Series RLC Load/LConn1
  Ideal Switch/LConn1 -- Battery +/RConn1 -- Battery1/LConn1 -- Battery3/LConn1 -- Ideal Switch2/LConn1 -- Battery2/LConn1 -- Ideal Switch1/LConn1
